simulink model "UnusedModels"  (R2015a)
settings: Solver=ode45  StartTime=0.0  StopTime=10.0  RelTol=1e-3
values from neighbouring files (symbols this model uses):
  car_params = Simulink_Car_params    [TV2016_parameters.m]
  energyLimitControl = Simulink_energyLimit    [TV2016_parameters.m]
  settings = Simulink_Settings    [TV2016_parameters.m]
  speedEstimation = Simulink_speedEst    [TV2016_parameters.m]
  tractionControl = Simulink_tc    [TV2016_parameters.m]
  yawRateControl = Simulink_yawRate    [TV2016_parameters.m]
undefined symbols (not defined in the file or in its folder): canChannel, Use_Estimated_velocity
libraries: canlib x44, CarMaker4SL x33, canmsglib x28, simulink x6
(part 4 of 4)

== matlab function UnusedModels/MATLAB Function ==
  data: Mz_ref input; Fx input; states input; Ti_lim output Bus: Ti_lim; Mz_error output; CM_Fxy input; car_params parameter; yaw_acc input; settings parameter; Mz output; R_eff_i input; Ti_prev input; Mz_calc output; Fz_ratio output; Fzi output; Long output; PseudoError output
function [Ti_lim, Mz_error,Mz,Mz_calc,Fz_ratio,Fzi,Long,PseudoError]= fcn(Mz_ref,Fx, states, CM_Fxy, car_params,yaw_acc,settings, R_eff_i, Ti_prev)
%#codegen


% % Splitte opp foran og bak-> vil hindre negativt moment på ytterhjul
% 
% %Fz scaling factor Calculation
% %The thought is 0 N Fz -> Cant use this wheel for torque
% % < 400N Fz , can use this wheel fully
% %Tire forces..
% Fzi = [states.Input_Fz_FL states.Input_Fz_FR states.Input_Fz_RL states.Input_Fz_RR]';
% 
% for i=1:4
%     if Fzi(i) <= 0
%         Fzi(i) = 1;
%     end
% end
% 
% dDt_Fz = 1/400;
% Fzi_Scaling = Fzi*dDt_Fz;
% for i=1:4
%     if ( Fzi_Scaling(i) < 0 )
%         Fzi_Scaling(i) = 0;
%     elseif (Fzi_Scaling(i) > 1)
%         Fzi_Scaling(i) = 1;
%     end
% end
% % 
% % % Scale all wheels with Fz first 
% % F_all = zeros(1,4);
% % %F_all = prod([Fx/4 Fx/4 Fx/4 Fx/4; Fzi_Scaling']);
% % F_all =[Fx/4 Fx/4 Fx/4 Fx/4];
% % % Find lateral split ratio
% % % Find longitudinal split ratio
% % 
% % if ((abs(r_ref)-abs(states.r)) <= 0)
% %     %Oversteering. Reduce torque on outer wheels
% %     ow_sf = 1- (1/settings.yaw_control_max_moment)*abs(Mz_ref);
% %     if sign(r_ref) == -1 
% %         %Right turn 
% %         F_all = prod([F_all;ow_sf 1 ow_sf 1]);
% %     else
% %         %Left turn
% %         F_all = prod([F_all;1 ow_sf 1 ow_sf]);
% %     end
% % else 
% %     %Find lateral split ratio
% %     l_sr = (1/settings.yaw_control_max_moment)*abs(Mz_ref);
% %     if sign(r_ref) == -1
% %         %Right turn
% %         F_all = prod([F_all;l_sr,(1-l_sr), l_sr, (1-l_sr)]);
% %     else 
% %         F_all = prod([F_all; (1-l_sr), l_sr , (1-l_sr) l_sr]);
% %     end
% % end
% 
% %Ratio between left and right wheels
% % Cases. 
% % 1. left turn r_ref larger than r. split more to outer wheels
% % 2. left turn r larger than r_ref. Reduce outher wheel torque
%     % Make scaling factor for outer wheels to reduce torque based on the Mz
% 
% % 3. right turn r_ref larger than r. split more to outer wheels
% % 4. right turn r larger than r_ref. Reduce outher wheel torque
%      % Make scaling factor for outer wheels to reduce torque based on the Mz
% 
% 
% 
% 
% %Calculate attainable torque for each motor
% Eng_rot_all = [Eng_rot.Eng_rot_FL Eng_rot.Eng_rot_FR Eng_rot.Eng_rot_RL Eng_rot.Eng_rot_RR];
% T_m_max = zeros(4,1);
% b = 20;
% a = -1/1000;
% x0 = 14000;
% for i=1:4
%     if Eng_rot_all(i) > 14000
%         T_m_max(i) = a*(Eng_rot_all(i)-x0) + b;
%     else 
%         T_m_max(i) = 21;
%     end
% end
% %Calculate allowable negative Torque limit
% T_m_neg = zeros(4,1);
% for i=1:4
%     if Fx == 0
%         T_m_neg(i) = 0;
%     elseif sign(Mz_ref) == sign(states.FL_Whl_Ang)
%         T_m_neg(i) = 0;
%     end
%     % Legge til at innerdekk ikke kan bruke negative torque eller positive
% end
% 
% 
% %1 = FL, 2 = FR, 3 = RL , 4 = RR
% R = [R_eff_i.R_FL; R_eff_i.R_FR ; R_eff_i.R_RL ; R_eff_i.R_RR]';
% 
% S = (states.FL_Whl_Ang + states.FR_Whl_Ang) / 2;
% l1 = car_params.t_f*cos(S) - car_params.l_f*sin(S);
% l2 = car_params.t_f*cos(S) + car_params.l_f*sin(S);
% l3 = car_params.t_r;
% l4 = car_params.t_r;
% 
% L = [-l1; l2; -l3; l4];  %*0.8;
% L_scaled = prod( [L'; Fzi'*settings.mui]);
% Tot_torque_scaled = prod( [1 1 1 1;Fzi'*settings.mui]);
% A_o = [L'; 1   1    1  1];
% %A = A*diag([Fzi'*settings.mui]);
% 
% %A = [L_scaled;Tot_torque_scaled]; %
% A = [L_scaled;Tot_torque_scaled
%     ]; % 
% 
% 
% %A_sat = diag([1 1 1 1]);
% 
% b = [Mz_ref; Fx];
% %Wu = diag([Fzi'*settings.mui]);
% Wu = diag( [1/Fzi(1)^2 1/Fzi(2)^2  1/Fzi(3)^2  1/Fzi(4)^2]);
%     
% 
%  
% Fx_i = zeros(4,1);
% %x is weighted by input
% %Fx_i = pinv(A)*b; %
% 
% 
% %Weighting by external weight matrix
% %Fx_i = Wu\(pinv(A/Wu))*b;
% Fx_i = inv(Wu)*A'*(inv(A*inv(Wu)*A'))*b
% %Fx_i = prod( [(pinv(A)*b)';Fzi_Scaling' ])';
% %Fx_i = (pinv(A)*b)
% PseudoError = A*Fx_i - b;
% Long = Tot_torque_scaled*Fx_i;
% 
% %x = (0,1)
% %Allocation based on Fz*x
% Ti_all = prod([Fx_i';R; Fzi'*settings.mui])*(1/settings.gear_ratio);
% Ti_lim_struct = struct;
% Ti_lim_struct.T_FL = Ti_all(1);
% Ti_lim_struct.T_FR = Ti_all(2);
% Ti_lim_struct.T_RR = Ti_all(4);
% Ti_lim_struct.T_RL = Ti_all(3);
% 
% 
% % Ti_all = prod([Fx_i';R])*(1/settings.gear_ratio)
% % Ti_lim_struct = struct;
% % Ti_lim_struct.T_FL = Ti_all(1);
% % Ti_lim_struct.T_FR = Ti_all(2);
% % Ti_lim_struct.T_RR = Ti_all(4);
% % Ti_lim_struct.T_RL = Ti_all(3);
% 
% Ti_lim = Ti_lim_struct; 
% 
% %Mz = -car_params.Iz * yaw_acc ; This is the total yaw moment which is not
% %what i am after.
% Mz = single(0); 
% Mz_calc = L_scaled*Fx_i;
% Mz_error = Mz_ref - Mz_calc;
% Fz_ratio = zeros(4,1);
% 
% for i=1:4
%     Fz_ratio(i,1) = sum( settings.mui^2*Fzi.^2 - Fx_i.^2) / (settings.mui^2*Fzi(i)^2 - Fx_i(i)^2);
% end

 
 %------------------------------------------------------------------------
 %------------------- Split Front/Rear------------------------------------
 %------------------------------------------------------------------------
 
% Splitte opp foran og bak-> vil hindre negativt moment på ytterhjul

%Fz scaling factor Calculation
%The thought is 0 N Fz -> Cant use this wheel for torque
% < 400N Fz , can use this wheel fully
%Tire forces..
Fzi = [states.Fz_FL states.Fz_FR states.Fz_RL states.Fz_RR]';

for i=1:4
    if Fzi(i) <= 0
        Fzi(i) = 1;
    end
end

dDt_Fz = 1/400;
Fzi_Scaling = Fzi*dDt_Fz;
for i=1:4
    if ( Fzi_Scaling(i) < 0 )
        Fzi_Scaling(i) = 0;
    elseif (Fzi_Scaling(i) > 1)
        Fzi_Scaling(i) = 1;
    end
end

%Calculate attainable torque for each motor
motor_RPMS = [states.RPM_FL states.RPM_FR  states.RPM_RL  states.RPM_RL]; 
T_m_max = zeros(4,1);
b = 20;
a = -1/1000;
x0 = 14000;
for i=1:4
    if motor_RPMS(i) > 14000
        T_m_max(i) = a*(motor_RPMS(i)-x0) + b;
    else 
        T_m_max(i) = 21;
    end
end
%Calculate allowable negative Torque limit
T_m_neg = zeros(4,1);
for i=1:4
    if Fx == 0
        T_m_neg(i) = 0;
    elseif sign(Mz_ref) == sign(states.FL_Whl_Ang)
        T_m_neg(i) = 0;
    end
    % Legge til at innerdekk ikke kan bruke negative torque eller positive
end


%1 = FL, 2 = FR, 3 = RL , 4 = RR
R = [R_eff_i.R_FL; R_eff_i.R_FR ; R_eff_i.R_RL ; R_eff_i.R_RR]';

S = (states.FL_Whl_Ang + states.FR_Whl_Ang) / 2;
l1 = car_params.t_f*cos(S) - car_params.l_f*sin(S); 
l2 = car_params.t_f*cos(S) + car_params.l_f*sin(S);
l3 = car_params.t_r;
l4 = car_params.t_r;

L = [-l1; l2; -l3; l4];  %*0.8;
L_scaled = prod( [L'; Fzi'*settings.mui]);
Tot_torque_scaled = prod( [1 1 1 1;Fzi'*settings.mui]);
A = [L_scaled;Tot_torque_scaled]; % 

A_f = [L_scaled(1) L_scaled(2);Tot_torque_scaled(1) Tot_torque_scaled(2)];
A_r = [L_scaled(3) L_scaled(4);Tot_torque_scaled(3) Tot_torque_scaled(4)];
%alfa_r = 0.5;

alfa_r =  (Fzi(3) + Fzi(4)) / (Fzi(1) + Fzi(2) +Fzi(3) + Fzi(4)); % How much of fz is at the rear..
b_f = [ (1-alfa_r) * Mz_ref; (1-alfa_r)*Fx];
b_r = [alfa_r*Mz_ref; alfa_r*Fx]; 


b = [Mz_ref; Fx];
%Wu = diag( [1/Fzi(1)^2 1/Fzi(2)^2  1/Fzi(3)^2  1/Fzi(4)^2]);
Wu_f = diag( [1/Fzi(1)^2 1/Fzi(2)^2]);
Wu_r = diag( [1/Fzi(3)^2 1/Fzi(4)^2]);

%u_f = zeros(2,1); % [-1,1] if over then it is saturated
%u_r = zeros(2,1); % [-1,1] 

Fx_i = zeros(4,1);
%x is weighted by input
%Fx_i = pinv(A)*b; %

%Weighting by external weight matrix
%Fx_i = Wu\(pinv(A/Wu))*b;

% u_f = Wu_f\pinv(A_f/Wu_f)*b_f
u_f2 = pinv(A_f)*b_f;
% u_r = Wu_r\pinv(A_r/Wu_r)*b_r;



%u_f = daisy_MzTot(u_f_pre,A_f,b_f,Wu_f);
%u_r = daisy_MzTot(u_r_pre,A_r,b_r,Wu_r);

% If sign(Mz) != turn allow negative torques for outer wheels
% Maybe if too high yaw rate only minimize Mz error.
% If not just use mz + tot(all positive)


% TRY THIS &
% Least squares for only Mz
% Then increase torque until saturation. But increase in which direction ?
A_mz_f = [A(1,1) A(1,2)];
A_mz_r = [A(1,3) A(1,4)];
b_mz_f = (1-alfa_r)*Mz_ref;
b_mz_r = alfa_r*Mz_ref;
u_f = single([0;0]);
u_r = single([0;0]);


u_f = distPseudoIterative_2State(A_f, b_f, states.r);
u_r = distPseudoIterative_2State(A_r, b_r, states.r);

%-------------------------------------------------%
%-----------Determine torque setpoints---------------%
%-------------------------------------------------%
Ti_all = prod([u_f' u_r';R; Fzi'*settings.mui])*(1/settings.gear_ratio);


Ti_lim_struct = struct;
Ti_lim_struct.T_FL = Ti_all(1);
Ti_lim_struct.T_FR = Ti_all(2);
Ti_lim_struct.T_RR = Ti_all(4);
Ti_lim_struct.T_RL = Ti_all(3);

Ti_lim = Ti_lim_struct; 



% if ( sign(Mz_ref) ~= sign(states.r) ) && abs(Mz_ref) > 30 && abs(states.r) > 1.3
% else
%     u_f = distPseudoIterative_2State(A_f, b_f, states.r);
%     u_r = distPseudoIterative_2State(A_r, b_r, states.r);
% end


% if one element of u_f is absolute > 1. 
% Find out which
% If only one, then saturate that input and solve equation for the other
% one.
% If that one saturates as well Finish (for now)
% If both saturated Finish (for now)


%u_f = inv(Wu_f)*A_f'*(inv(A_f*inv(Wu_f)*A_f'))*b_f;
%u_r = inv(Wu_r)*A_r'*(inv(A_r*inv(Wu_r)*A_r'))*b_r;


%-----------------------------------
%-------Allokering med vekt artikkel---

u_opt_f = (Wu_f + A_f'*A_f)\A_f'*b_f;
%u_f = [0;0];
%u_f = pinv(A_f)*b_f;
%u_r = pinv(A_r)*b_r

%Fx_i = inv(Wu)*A'*(inv(A*inv(Wu)*A'))*b
%Fx_i = prod( [(pinv(A)*b)';Fzi_Scaling' ])';
%Fx_i = (pinv(A)*b)

%x = (0,1)
%Allocation based on Fz*x


%Ti_all = prod([Fx_i';R; Fzi'*settings.mui])*(1/settings.gear_ratio);





%Mz = -car_params.Iz * yaw_acc ; This is the total yaw moment which is not
%what i am after.

PseudoError = single(0); % A*Fx_i - b;
Long = single(0); % Tot_torque_scaled*Fx_i;

Mz = single(0); 
Mz_calc = L_scaled*[u_f;u_r];
Mz_error = Mz_ref - Mz_calc;
%Mcalc = L'*(prod([Ti_all';1./R])*GR)';
%Mz_error = Mz_ref - Mcalc;

Fz_ratio = zeros(4,1);

for i=1:4
    Fz_ratio(i,1) = sum( settings.mui^2*Fzi.^2 - Fx_i.^2) / (settings.mui^2*Fzi(i)^2 - Fx_i(i)^2);
end
end


function u_x = daisy_Mz(u_in,A,b)
    u_x = single(zeros(2,1));
    l = u_in(1);
    r = u_in(2);
    if ( abs(l) > 1) && ( abs(r) <= 1) 
        %W = W(2,2); % Second input should be weighted
        A_x = A(1,2)
        b_new = b - sign(l)*A(1,1);
        r = pinv(A_x)*b_new;
        l = 1*sign(l);
        u_x = [l;r];
    elseif ( abs(r) > 1) && ( abs(l) <= 1)
        %W = W(1,1); % First input should be weighted
        A_x = A(1,1);
        b
        b_new = b - sign(r)*A(1,2)
        l = pinv(A_x)*b_new
        r = 1*sign(r)
        u_x = [l;r]
        error = A*u_x - b    
        % Kommer ut av daisy med negativ torque på ene hjulet-> vanlig
        % pseudo liker det dårlig( fx + fx = tot_fx).. blir ustabilt.
    elseif ( abs(r) > 1) && ( abs(l) > 1)
        %Solve for both, then choose the best
        
        u_x = [sign(l);sign(r)];
        
        hoi = 5
    else 
        u_x = u_in;
    end
end

function u = distPseudoIterative(B_in, tau,nr_u_solved,u_size)
    % B = A, tau = b
    coder.varsize('B',[2,4]);
    coder.varsize('u_sat',[4,1]);
    coder.varsize('B_sat',[2,4]);
    coder.varsize('B_unsat',[2,4]);
    B = B_in;
    u_solved = single(-10*ones(u_size,1));
%     u_sat   = zeros(4,1);
%     B_sat   = zeros(2, 4);
%     B_unsat = zeros(2, 4);
    for z=1:10
        z
        [row_B,col_B] = size(B);
        row_tau = row_B;
        u_1 = pinv(B)*tau
        %Find number of saturated elements
        nr_sat_elements = 0;
        for i=1:col_B
            if abs(u_1(i)) > 1
                nr_sat_elements = nr_sat_elements + 1;
            end
        end
        if (nr_sat_elements == 0) 
            open_spot_counter = 0;
            % Must fill in u_1 into u_solved...
            if nr_u_solved == 0
                % If solved on first attempt fit u_1 into u solved and
                % return
                u = u_1;
                return  
            else
                % Not first attempt, then need to fill in u_1 into u_solved
                for i=1:size(u_1,1)
                    for a=1:u_size
                        if u_solved(a) == -10
                            open_spot_counter = open_spot_counter + 1;
                            if open_spot_counter == i 
                                u_solved(a) = sign(u_1(i));
                                break
                            end
                        end
                    end
                end   
                u = u_solved;
                return
            end   
        end
        %Split into saturated and non saturated
        
%         if (nr_sat_elements == 1)
%             u_sat = 0;
%             B_sat = zeros(row_B,1);
%             B_unsat = zeros(row_B, col_B - 1);
%         elseif (nr_sat_elements == 2)
%             u_sat = zeros(2,1);
%             B_sat = zeros(row_B,2);
%             B_unsat = zeros(row_B, col_B - 2);
% 
%         elseif (nr_sat_elements == 3)
%             u_sat = zeros(3,1);
%             B_sat = zeros(row_B,3);
%             B_unsat = zeros(row_B, col_B - 3);
% 
%         elseif (nr_sat_elements == 4)
%             u_sat = zeros(4,1);
%             B_sat = zeros(row_B,4); 
%             B_unsat = zeros(1,1);
% 
%         else
%             B = zeros(row_B,1);
%             u_sat = 0;
%             B_sat = zeros(row_B,1); 
%         end
        
        assert(nr_sat_elements < 5);
        u_sat   = zeros(nr_sat_elements,1);
        B_sat   = zeros(row_B, nr_sat_elements);
        B_unsat = zeros(row_B, col_B - nr_sat_elements);
        sat_counter     = 1;
        unsat_counter   = 1;
        open_spot_counter = 0;
        for i=1:col_B
            if abs(u_1(i)) > 1
                u_sat(sat_counter) = sign(u_1(i));
                %Fill in new saturated elements into the solution vector
                % Need to add the elements
                if col_B == u_size
                    u_solved(i) = sign(u_1(i));
                else              
                    %Search for first open spot corresponding with i
                    for a=1:u_size
                        if u_solved(a) == -10
                            open_spot_counter = open_spot_counter + 1;
                            if open_spot_counter == i 
                                u_solved(a) = sign(u_1(i))
                                break
                            end
                            
                        end
                    end
                end
                
                nr_u_solved = nr_u_solved + 1;
                for j=1:row_B
                    B_sat(j, sat_counter) = B(j,i);
                end  
                sat_counter = sat_counter + 1;
            elseif abs(u_1(i)) <= 1
                for j=1:row_B
                    B_unsat(j, unsat_counter) = B(j,i);
                end
                unsat_counter = unsat_counter + 1;
            else
                thisShouldNotHappen = 1
            end

        end
        % Now I have saturated B and u and unsaturated B
        tau = tau - B_sat*u_sat;
        B = single(B_sat);
%         B = zeros(size(B_sat,1),size(B_sat,2))
%         for i=1:size(B_sat,1)
%             for j=1:size(B_sat,2)
%                 B(i,j) = B_sat(i,j);
%             end
%         end
        
        %Now I have the new problem
        if nr_u_solved == u_size 
            u = u_solved;
            return
        end
    end
    u = u_solved;
end
    



function u_x = daisy_MzTot(u_in,A,b,W)
    u_x = single(zeros(2,1));
    l = u_in(1);
    r = u_in(2);
    if ( abs(l) > 1) & ( abs(r) <= 1) 
        W = W(2,2); % Second input should be weighted
        A_x = [ A(1,2);A(2,2)];
        b_new = b - sign(l)*[A(1,1);A(2,1)];
        r = pinv(A_x)*b_new;
        l = 1*sign(l);
        u_x = [l;r];
    elseif ( abs(r) > 1) & ( abs(l) <= 1)
        W = W(1,1); % First input should be weighted
        A_x = [ A(1,1);A(2,1)]
        b
        b_new = b - sign(r)*[A(1,2);A(2,2)]
        l = pinv(A_x)*b_new
        r = 1*sign(r)
        u_x = [l;r]
        error = A*u_x - b    
        % Kommer ut av daisy med negativ torque på ene hjulet-> vanlig
        % pseudo liker det dårlig( fx + fx = tot_fx).. blir ustabilt.
    elseif ( abs(r) > 1) & ( abs(l) > 1)
        %Solve for both, then choose the best
        u_x = [sign(l); sign(r)]
        hoi = 5
    else 
        u_x = u_in;
    end
end
%u_f = Wu_f\pinv(A_f/Wu_f)*b_f

function u = distPseudoIterative_2State(B, tau, r)
    u_1 = pinv(B)*tau;
    if ( abs(u_1(1)) <= 1 && abs(u_1(2)) <= 1 )
        % None saturated. Return
        u = u_1;
        return
    elseif ( abs(u_1(1)) > 1 && abs(u_1(2)) <= 1 )
        % Nr 1 saturated
        B_sat = [B(1,1);B(2,1)];
        B_unsat = [B(1,2);B(2,2)];
        tau_proj = tau - B_sat*(sign(u_1(1)));
        right = pinv(B_unsat)*tau_proj;
        if abs(right) > 1 
            right = sign(right);
        end

        u = [sign(u_1(1));right]; 
        % Do something if u is also saturated
        return

    elseif ( abs(u_1(1)) <= 1 && abs(u_1(2)) > 1 )
         % Nr 2 saturated
        B_sat = [B(1,2);B(2,2)];
        B_unsat = [B(1,1);B(2,1)];
        tau_proj = tau - B_sat*(sign(u_1(2)));
        left = pinv(B_unsat)*tau_proj;
        if abs(left) > 1 
            left = sign(left);
        end   
        u = [left;sign(u_1(2))]; 
        % Do something if u is also saturated
        return

    elseif ( abs(u_1(1)) > 1 && abs(u_1(2)) > 1 )
        % If turning right input 1 should be saturated and input 2
        % recomputed
        %If turning left opposite

        if ( sign(r) == 1)
            %turning left, right wheel saturate
            B_sat = [B(1,2);B(2,2)];
            B_unsat = [B(1,1);B(2,1)];
            tau_proj = tau - B_sat*(sign(u_1(2)));
            left = pinv(B_unsat)*tau_proj;
            if abs(left) > 1 
                left = sign(left);
            end   
            u = [left;sign(u_1(2))];
            return
        elseif (sign(r) == -1)
            %turning right
            % Nr 1 saturated
            B_sat = [B(1,1);B(2,1)];
            B_unsat = [B(1,2);B(2,2)];  
            tau_proj = tau - B_sat*(sign(u_1(1)));
            right = pinv(B_unsat)*tau_proj;
            if abs(right) > 1 
                right = sign(right);
            end
            u = [sign(u_1(1));right]; 
            % Do something if u is also saturated
            return
        else
            %Not turning
            %Saturate both and return
            u = [sign(u_1(1));sign(u_1(2))];  
            return
        end
    else
        u = u_1;
        return
    end
end

== matlab function UnusedModels/Estimations /RPM to wheel x velocities/Calculate velocity of each wheel ==
  data: sensor input; Whl_v_FL output; Whl_v_FR output; Whl_v_RL output; Whl_v_RR output; settings parameter; car_params parameter
function [Whl_v_FL, Whl_v_FR, Whl_v_RL, Whl_v_RR]  = RpmToVelocity(sensor,settings,car_params)
%#codegen

%Conversion from RPM to rad/s for the wheel
c = single(2*pi/(car_params.GR*60));

% Simple atm. Not considering rotation and vy
Whl_v_FL = sensor.RPM_FL*c*car_params.r_eff;
Whl_v_FR = sensor.RPM_FR*c*car_params.r_eff;
Whl_v_RL = sensor.RPM_RL*c*car_params.r_eff;
Whl_v_RR = sensor.RPM_RR*c*car_params.r_eff;

== matlab function UnusedModels/SimpleTv/MATLAB Function ==
  data: muR input; Ti_lim output Bus: Ti_lim; Fx input; states input; settings parameter; R_eff_i input; car_params parameter; Mz_ref input; Ti_max output; Mz_error output
function [Ti_lim,Ti_max,Mz_error]  = fcn(muR,Fx,states,settings,R_eff_i, car_params,Mz_ref )
%#codegen
%STATES
r = states.r;

%PARAMETERS
mu = settings.mui;
tf = car_params.t_f*2;
tr = car_params.t_r*2;
GR = car_params.GR;
R = [R_eff_i.R_FL; R_eff_i.R_FR ; R_eff_i.R_RL ; R_eff_i.R_RR]';
%Load Transfer
Fzi = [states.Fz_FL states.Fz_FR states.Fz_RL states.Fz_RR]';
alfa_r =  (Fzi(3) + Fzi(4)) / (Fzi(1) + Fzi(2) +Fzi(3) + Fzi(4)); 






%FIND MAXIMUM ALLOWED MOTOR TORQUE, TIRE/MOTOR
Ti_max          = single(zeros(4,1));
Ti_max_tire     = single(zeros(4,1));
Ti_max_motor    = single(zeros(4,1));

RPM = [states.RPM_FL, states.RPM_FR, states.RPM_RL, states.RPM_RR];
a = 8/7000;
a2 = 13/1000;
for i=1:4
    if RPM(i) >= 20000 
        Ti_max_motor(i) = 0;
    elseif RPM(i) > 12000 & RPM(i) < 19000
        Ti_max_motor(i) = -a*(RPM(i) - 12000) + 21;
    elseif RPM(i) > 19000 & RPM(i) < 20000
        Ti_max_motor(i) = -a2*(RPM(i) - 19000) + 13;
    else 
        Ti_max_motor(i) = 21;
    end
end
%Tire saturation based on mu and Fz
for i=1:4
    Ti_max_tire(i) = Fzi(i)*mu*R(i)/GR;
end
% Find minimum of tire saturation Torque and motor
for i=1:4
    Ti_max(i) = min(Ti_max_tire(i), Ti_max_motor(i));
end
%**********************************************%

T_F = single(zeros(2,1));
T_R = single(zeros(2,1));

T_F = dist(Ti_max(1), Ti_max(2), Fx, R(1), R(2), (1-alfa_r), Mz_ref, GR, tf);
T_R = dist(Ti_max(3), Ti_max(4), Fx, R(3), R(4), alfa_r, Mz_ref, GR, tr);


% T_FL = (1-alfa_r)*Fx*R(1)/(2*GR) - (1-alfa_r)*Mz_ref*R(1)/(GR*tf);
% T_FR = (1-alfa_r)*Fx*R(2)/(2*GR) + (1-alfa_r)*Mz_ref*R(2)/(GR*tf);
% T_RL = (alfa_r)*Fx*R(3)/(2*GR) - alfa_r*Mz_ref*R(3)/(GR*tr);
% T_RR = (alfa_r)*Fx*R(4)/(2*GR) + alfa_r*Mz_ref*R(4)/(GR*tr);

%Ti_all = [T_FL, T_FR, T_RL, T_RR];
Ti_all = [T_F' T_R'];

Ti_lim_struct = struct;
Ti_lim_struct.T_FL = Ti_all(1);
Ti_lim_struct.T_FR = Ti_all(2);
Ti_lim_struct.T_RR = Ti_all(4);
Ti_lim_struct.T_RL = Ti_all(3);

Ti_lim = Ti_lim_struct;



% Mz_error Calc

S = states.steering_angle;
l1 = car_params.t_f*cos(S) - car_params.l_f*sin(S); 
l2 = car_params.t_f*cos(S) + car_params.l_f*sin(S);
l3 = car_params.t_r;
l4 = car_params.t_r;

L = [-l1; l2; -l3; l4];
Fx_all = prod([Ti_all; 1./R;])*GR;
Mz_allocated = L'*Fx_all';
Mz_error = Mz_ref - Mz_allocated;


end

function T = dist(L_max, R_max, Fx, R_eff_L, R_eff_R, alfa, Mz_ref, GR, t )
    T = single(zeros(2,1));
    L = alfa*Fx*R_eff_L/(2*GR) - alfa*Mz_ref*R_eff_L/(GR*t);
    R = alfa*Fx*R_eff_R/(2*GR) + alfa*Mz_ref*R_eff_R/(GR*t);

    if ( abs(L) <=  L_max) && ( abs(R) <= R_max)
        % None are saturated. Return
        T = [L;R];
        return
    elseif abs(L) > L_max && abs(R) < R_max
        % Left is saturated
        % How much?
        Sat_amount = abs(L) - L_max;
        L = L - sign(L)*Sat_amount;
        R = R - sign(R)*Sat_amount;
        T = [L;R];
        return;
    elseif abs(R) > R_max && abs(L) < L_max
        Sat_amount = abs(R) - R_max;
        L = L - sign(L)*Sat_amount;
        R = R - sign(R)*Sat_amount;
        T = [L;R];
        return;
    elseif (abs(R) > R_max) && (abs(L) > L_max)
        %Which is the most saturated?
        Sat_amount = max( (abs(L) - L_max), (abs(R)- R_max));
        L = L - sign(L)*Sat_amount;
        R = R - sign(R)*Sat_amount;
        T = [L;R];
        return;
    else
        T = [L;R];
        return
    end
end

== matlab function UnusedModels/Function-Call Subsystem/MATLAB Function ==
  data: trq_pos_16 input; trq_pos_f output; trq_neg_16 input; w_set_16 input; trq_neg_f output; w_set_f output; settings parameter
function [trq_pos_f, trq_neg_f, w_set_f] = fcn(trq_pos_16, trq_neg_16, w_set_16, settings)
%#codegen

Sf = settings.scaling_factor;
trq_pos_f = double( trq_pos_16/Sf);
trq_neg_f = double( trq_neg_16/Sf);
w_set_f = double( w_set_16);

== matlab function UnusedModels/Estimations /Normal Force Direct Calculation/MATLAB Function ==
  data: sensor input; settings parameter; car_params parameter; Fz_FL output; Fz_FR output; Fz_RL output; Fz_RR output
function [Fz_FL, Fz_FR, Fz_RL, Fz_RR] = normalForceEstimation(sensor, settings,car_params)
%#codegen

te = settings.control_system_sample_time;
ms = car_params.sprung_mass; 
mv = car_params.mass; % Total mass( driver + car)
l = car_params.l; %Wheel base
lr = car_params.l_r;
lf = car_params.l_f;
hr = car_params.h_r;
hf = car_params.h_f;
tf = car_params.t_f*2; % Front track
tr = car_params.t_r*2; % Rear track
kf = car_params.roll_stiff_f;
kr = car_params.roll_stiff_r;
Ixx = car_params.Ixx;
hcr = car_params.h_cr;
Kr = car_params.K_r;
Cr = car_params.C_r;
hc = car_params.CoG_height;
g = 9.81;

ax = sensor.ax;
ay = sensor.ay;

Fz_FL = 0.5*mv*(lr*g/l - hc*ax/l) - mv*(lr*g/l - hc*ax/l) * hc*ay/(tf*g);

Fz_FR = 0.5*mv*(lr*g/l - hc*ax/l) + mv*(lr*g/l - hc*ax/l) * hc*ay/(tf*g);

Fz_RL = 0.5*mv*(lf*g/l + hc*ax/l) - mv*(lf*g/l + hc*ax/l) * hc*ay/(tr*g);

Fz_RR = 0.5*mv*(lf*g/l + hc*ax/l) + mv*(lf*g/l + hc*ax/l) * hc*ay/(tr*g);




end

== matlab function UnusedModels/Function-Call Subsystem1/MATLAB Function1 ==
  data: trq_pos_16 input; trq_pos_f output; trq_neg_16 input; w_set_16 input; trq_neg_f output; w_set_f output; settings parameter
function [trq_pos_f, trq_neg_f, w_set_f] = fcn(trq_pos_16, trq_neg_16, w_set_16, settings)
%#codegen

Sf = settings.scaling_factor;
trq_pos_f = double( trq_pos_16/Sf);
trq_neg_f = double( trq_neg_16/Sf);
w_set_f = double( w_set_16);

== matlab function UnusedModels/Function-Call Subsystem3/MATLAB Function3 ==
  data: trq_pos_16 input; trq_pos_f output; trq_neg_16 input; w_set_16 input; trq_neg_f output; w_set_f output; settings parameter
function [trq_pos_f, trq_neg_f, w_set_f] = fcn(trq_pos_16, trq_neg_16, w_set_16, settings)
%#codegen

Sf = settings.scaling_factor;
trq_pos_f = double( trq_pos_16/Sf);
trq_neg_f = double( trq_neg_16/Sf);
w_set_f = double( w_set_16);

== matlab function UnusedModels/Function-Call Subsystem2/MATLAB Function2 ==
  data: trq_pos_16 input; trq_pos_f output; trq_neg_16 input; w_set_16 input; trq_neg_f output; w_set_f output; settings parameter
function [trq_pos_f, trq_neg_f, w_set_f] = fcn(trq_pos_16, trq_neg_16, w_set_16, settings)
%#codegen

Sf = settings.scaling_factor;
trq_pos_f = double( trq_pos_16/Sf);
trq_neg_f = double( trq_neg_16/Sf);
w_set_f = double( w_set_16);

== matlab function UnusedModels/Estimations /Subsystem/Compute Derivative of RPM ==
  data: RPM_FL input; rateRPM_FL output; RPM_FR input; RPM_RL input; RPM_RR input; settings parameter; rateRPM_FR output; rateRPM_RL output; rateRPM_RR output
function [rateRPM_FL,rateRPM_FR,rateRPM_RL,rateRPM_RR]...
          = computeRPMDerivative(RPM_FL,RPM_FR,RPM_RL,RPM_RR,settings)
%#codegen

t = settings.control_system_sample_time;
sg_Weight = single( [ -1; 8; 0; -8; 1] );

nr_Coefficients = uint32(5);
persistent firstIteration;
persistent frame;
persistent RPM_prev_FL;
persistent RPM_prev_FR;
persistent RPM_prev_RL;
persistent RPM_prev_RR;


if isempty(firstIteration)
        firstIteration = 2;
        RPM_prev_FL = RPM_FL;
        RPM_prev_FR = RPM_FR;
        RPM_prev_RL = RPM_RL;
        RPM_prev_RR = RPM_RR;
        
        frame = single(zeros(1,nr_Coefficients));
        rateRPM_FL = single(0);
        rateRPM_FR = single(0);
        rateRPM_RL = single(0);
        rateRPM_RR = single(0);
else
    rateRPM_FL = abs( (RPM_FL - RPM_prev_FL)/(t));
    rateRPM_FR = abs( (RPM_FR - RPM_prev_FR)/(t));
    rateRPM_RL = abs( (RPM_RL - RPM_prev_RL)/(t));
    rateRPM_RR = abs( (RPM_RR - RPM_prev_RR)/(t));
    RPM_prev_FL = RPM_FL;
    RPM_prev_FR = RPM_FR;
    RPM_prev_RL = RPM_RL;
    RPM_prev_RR = RPM_RR;
    
    
%     frame = [RPM, frame(1:(end-1))]    
%     %Calculate output
%     rateRPM = abs((frame*weight_Vector)./(12*ts));


end

== matlab function UnusedModels/Function-Call Subsystem4/MATLAB Function ==
  data: trq_pos_16 input; trq_pos_f output; trq_neg_16 input; w_set_16 input; trq_neg_f output; w_set_f output; settings parameter
function [trq_pos_f, trq_neg_f, w_set_f] = fcn(trq_pos_16, trq_neg_16, w_set_16, settings)
%#codegen

Sf = settings.scaling_factor;
trq_pos_f = double( trq_pos_16/Sf);
trq_neg_f = double( trq_neg_16/Sf);
w_set_f = double( w_set_16);

== matlab function UnusedModels/Function-Call Subsystem4/MATLAB Function1 ==
  data: trq_pos_16 input; trq_pos_f output; trq_neg_16 input; w_set_16 input; trq_neg_f output; w_set_f output; settings parameter
function [trq_pos_f, trq_neg_f, w_set_f] = fcn(trq_pos_16, trq_neg_16, w_set_16, settings)
%#codegen

Sf = settings.scaling_factor;
trq_pos_f = double( trq_pos_16/Sf);
trq_neg_f = double( trq_neg_16/Sf);
w_set_f = double( w_set_16);

== matlab function UnusedModels/Function-Call Subsystem4/MATLAB Function2 ==
  data: trq_pos_16 input; trq_pos_f output; trq_neg_16 input; w_set_16 input; trq_neg_f output; w_set_f output; settings parameter
function [trq_pos_f, trq_neg_f, w_set_f] = fcn(trq_pos_16, trq_neg_16, w_set_16, settings)
%#codegen

Sf = settings.scaling_factor;
trq_pos_f = double( trq_pos_16/Sf);
trq_neg_f = double( trq_neg_16/Sf);
w_set_f = double( w_set_16);

== matlab function UnusedModels/Function-Call Subsystem4/MATLAB Function3 ==
  data: trq_pos_16 input; trq_pos_f output; trq_neg_16 input; w_set_16 input; trq_neg_f output; w_set_f output; settings parameter
function [trq_pos_f, trq_neg_f, w_set_f] = fcn(trq_pos_16, trq_neg_16, w_set_16, settings)
%#codegen

Sf = settings.scaling_factor;
trq_pos_f = double( trq_pos_16/Sf);
trq_neg_f = double( trq_neg_16/Sf);
w_set_f = double( w_set_16);

== matlab function UnusedModels/Fz_Estimation/FzEst ==
  data: normalForces output Bus: normalForces; sensor input; settings parameter; car_params parameter; x_out output; xv_out output; FZ output; delta_Fzl output
function [normalForces, x_out,xv_out,FZ,delta_Fzl] = normalForceEstimation(sensor, settings,car_params)
%#codegen

te = settings.control_system_sample_time;

ms = car_params.sprung_mass; 
mv = car_params.mass; % Total mass( driver + car)
l = car_params.l; %Wheel base
lr = car_params.l_r;
lf = car_params.l_f;
hr = car_params.h_r;
hf = car_params.h_f;
ef = car_params.t_f*2; % Front track
er = car_params.t_r*2; % Rear track
kf = car_params.roll_stiff_f;
kr = car_params.roll_stiff_r;
Ixx = car_params.Ixx;
hcr = car_params.h_cr;
Kr = car_params.K_r;
Cr = car_params.C_r;
hc = car_params.CoG_height;
g = 9.81;


%ODFzL = linear lateral
%OFzE = nonlinear vertical
%OFzL = linear vertical


%State vector
A = zeros(5,5);
H = zeros(5,5);
A = single([1 0 -2*te*(ms/l)*( (lr*hf)/ef + (lf*hr)/er) 0 -2*te*(kf/ef + kr/er);
     0 1 te 0 0;
     0 0 1 0 0;
     0 0 0 1 te;
     0 te*ms*hcr/Ixx 0 te*(ms*g*hcr - Kr)/Ixx  (1+te*(-Cr)/Ixx)]);
%Only use roll rate measurement
%A = single([1 0 -2*te*(ms/l)*( (lr*hf)/ef + (lf*hr)/er) 0 -2*te*(kf/ef + kr/er);
%    0 1 te 0 0;
%    0 0 1 0 0;
%    0 0 0 1 te;
%    0 0 0 0 0]);

% PS: If we measure true linear compensated ay, we dont need to
% adjust with roll angle or gravity. Just double check this.
H = single([0 1 0 0 0;
    0 0 0 1 0;
    0 0 0 0 1;
    1 0 0 0 0]);
%-------------------------------------------------------%
%-------------------------Lateral LKF-------------------%
%-------------------------------------------------------%
persistent firstIteration;
persistent x;
persistent P;

%State Vector: x = [left load transfer , ay_k , der_ay_k , rollAngle, rollRate]
%Measurement vector = [aym, rollAngle, rollRate, left load transfer meas]

%Q = single(diag([1000, 0.1, 0.1, 0.1, 0.1])); % Book parameters
% Notice that last state is weighted very low since there is no process
Q = single(diag([1000, 0.1, 0.1, 0.1, 0.001])); % Book parameters

R = single( diag([0.01 0.01 0.01 100])); % Taken from book

K = single(zeros(5,4));

x_out = single(zeros(5,1));
delta_Fzl = single(0);
if isempty(firstIteration)
    %firstIteration = 2; % Avoid overflow in the register and count 1 again
    %First time the function is called
    %Initialize
    P = single(eye(5));
    x = single(zeros(5,1)); % Also initial value
    x_out = x;
else
	x = A*x; % Prediction of the state
    P = A*P*A' + Q; % Predicted covariance
    
    %Measurement Update
    K = P*H'*inv(H*P*H' + R); % The filter gain
    Y_predicted = H*x; % Predicted measurement
    
    delta_Fzl = -2*(kf/ef + kr/er)*sensor.roll_angle - 2*ms*(sensor.ay/l)*(lr*hf/ef + lf*hr/er);
    Y_meas      = [sensor.ay; sensor.roll_angle; sensor.roll_rate; delta_Fzl];
    
    e = Y_meas - Y_predicted; %Difference between the measurement and predicted measurement 
    x = x + K*e; % Corrected state estimate
    x_out = x;
    P = P - K*H*P;
end

%-------------------------------------------------------%
%-------------------------Vertical Force LKF------------%
%-------------------------------------------------------%
%Assumes superposition principle. Change from LKF to EKF when time
a = te*(-mv*hc)/(2*l);
b = te*(-lr*mv*hc)/(l*ef);
br = te*(-lf*mv*hc)/(l*er);
Av = single([1 0 0 0 0 a 0 b;
            0 1 0 0 0 a 0 -b;
            0 0 1 0 0 -a 0 br;
            0 0 0 1 0 -a 0 -br;
            0 0 0 0 1 te 0 0;
            0 0 0 0 0 1 0 0;
            0 0 0 0 0 0 1 te;
            0 0 0 0 0 0 0 1]);
Hv = single([1 -1 1 -1 0 0 0 0;
            1 1 0 0 0 0 0 0;
            0 0 0 0 1 0 0 0;
            0 0 0 0 0 0 1 0;
            1 1 1 1 0 0 0 0]);
persistent xv;
persistent Pv;


Qv = single(diag([100 100 100 100 0.1 0.001 0.1 0.001])); % From book
Rv = single(diag([0.1 100 0.01 0.01 100])); % Taken from book( VehicleDynest)
Kv = single(zeros(8,5));      % Kalman gain

xv_out = single(zeros(8,1));
Y_measv = single(zeros(5,1));
Y_predictedv = single(zeros(5,1));

%-----------------------------------
%Normal force each tire calculcation
%-----------------------------------
%-----------------------------------
%Normal force each tire calculcation 2
%-----------------------------------
Fz11 = 0.5*mv*(lr*g/l - hc*sensor.ax/l) - mv*(lr*g/l - hc*sensor.ax/l)*hc*sensor.ay/(ef*g);
Fz12 = 0.5*mv*(lr*g/l - hc*sensor.ax/l) + mv*(lr*g/l - hc*sensor.ax/l)*hc*sensor.ay/(ef*g);

Fz21 = 0.5*mv*(lf*g/l + hc*sensor.ax/l) - mv*(lf*g/l + hc*sensor.ax/l)*hc*sensor.ay/(er*g);
Fz22 = 0.5*mv*(lf*g/l + hc*sensor.ax/l) + mv*(lf*g/l + hc*sensor.ax/l)*hc*sensor.ay/(er*g);

FZ = [Fz11; Fz12; Fz21; Fz22];

% Output:
Fz_FL = single(0);
Fz_FR = single(0);
Fz_RL = single(0);
Fz_RR = single(0);



% qf1 = 0.5*mv*(lr*g/l - hc*sensor.a_x/l);
% qf2 = mv*(lr*g/l - hc*sensor.a_x/l)*hc*sensor.a_y/(ef*g);
% Fz11 = qf1 - qf2; % sensor a_y or estimated a_y ????
% Fz12 = qf1 + qf2;
%FzObs = single(mv*(lr*g/l - hc*sensor.ax/l));

normalForces.FL = single(0);
normalForces.FR = single(0);
normalForces.RL = single(0);
normalForces.RR = single(0);

FzObs = single( Fz11 + Fz12);
mxx = single(mv*g/4);
sum_Fz = single(mv*g);
if isempty(firstIteration)
    firstIteration = 2; % Avoid overflow in the register and count 1 again
    %First time the function is called
    %Initialize
    xv = [mxx; mxx; mxx; mxx; 0; 0; 0; 0];
    Pv = single(eye(8));
    xv_out = xv;   
else
	xv = Av*xv; % Prediction of the state
    Pv = Av*Pv*Av' + Qv; % Predicted covariance
    
    %Measurement Update
    Kv = Pv*Hv'/(Hv*Pv*Hv' + Rv); % The filter gain
    Y_predictedv = Hv*xv; % Predicted measurement
    
    Y_measv      = [x(1); FzObs; sensor.ax; x(2); sum_Fz];
    %x(1) = delta_Fzl from other observer
    %x(2) = estimated lateral acceleration compensating for roll angle
    ev = Y_measv - Y_predictedv; %Difference between the measurement and predicted measurement 
    xv = xv + Kv*ev; % Corrected state estimate
    xv_out = xv;
    Pv = Pv - Kv*Hv*Pv;
    normalForces.FL = xv_out(1);
    normalForces.FR = xv_out(2);
    normalForces.RL = xv_out(3);
    normalForces.RR = xv_out(4);
%     Fz_FL = xv_out(1);
%     Fz_FR = xv_out(2);
%     Fz_RL = xv_out(3);
%     Fz_RR = xv_out(4);
    
    
end

== matlab function UnusedModels/Slip ratio ==
  data: SR_Kp output; SR_Ki output; SR_ref output; states input; tractionControl parameter; SR_FL output; SR_FR output; SR_RL output; SR_RR output; speed output
function [SR_Kp, SR_Ki, SR_ref, SR_FL, SR_FR, SR_RL, SR_RR, speed] = slipRatioCalculation(states,tractionControl)
%#codegen
SR_ref = single(tractionControl.Slip_ratio_ref);

SR_FL = single((states.whl_v_FL - states.V_x) / max([0.01, abs(states.whl_v_FL), abs(states.V_x)]));
SR_FR = single((states.whl_v_FR - states.V_x) / max([0.01, abs(states.whl_v_FR), abs(states.V_x)]));
SR_RL = single((states.whl_v_RL - states.V_x) / max([0.01, abs(states.whl_v_RL), abs(states.V_x)]));
SR_RR = single((states.whl_v_RR - states.V_x) / max([0.01, abs(states.whl_v_RR), abs(states.V_x)]));




% GAIN SCHEDULING

%Kp = some function of v_x
%Ki = some function of v_x

SR_Kp = tractionControl.Kp;
SR_Ki = tractionControl.Ki;

speed = states.V_x;
% if (states.V_x < 1) 
%     SR_Kp = single(5);
%     SR_Ki = single(0);
% else
%     SR_Kp = single(5);
%     SR_Ki = single(200);
% end

end

== matlab function UnusedModels/Energy limit Torque Reduction Controller/Energy Limit Control ==
  data: average_power output; states input; energyLimitControl parameter
function average_power  = energyLimitControl(states,energyLimitControl)
%#codegen


%persistent energy;
persistent powerCounter;
persistent firstIteration;
persistent accumulatedTime;
persistent nr_Samples;


if isempty(firstIteration)
    firstIteration = 2; 
    powerCounter = single(0);
    average_power = powerCounter;
    accumulatedTime = single(0);
    
    nr_Samples = single(0);
else
    if (states.power < 0)
        nr_Samples = nr_Samples + single(1);
        powerCounter =  (abs(states.power) + nr_Samples*powerCounter) / (nr_Samples + 1);
        accumulatedTime = accumulatedTime + energyLimitControl.time_since_last_value;
        if (accumulatedTime > energyLimitControl.time_frame)            
            average_power = powerCounter;
        else
            average_power = single(0);
        end 
    else
        nr_Samples = single(0);
        accumulatedTime = single(0);
        powerCounter = single(0);
        average_power = single(0);

    end
end
end

    
    
    

%     
% if (states.effect < 0)
%     energy = energy + abs(energyLimitControl.time_since_last_value*states.effect);
%     accumulated_energy = energy;
% else
%     energy = single(0);
%     accumulated_energy = energy;
% end

== matlab function UnusedModels/FzEstCoupledKalmanFilters ==
  data: normalForces output Bus: normalForces; sensor input Bus: SensorInputs; settings parameter; car_params parameter; x_out output; xv_out output; FZ output; delta_Fzl output
function [normalForces, x_out,xv_out,FZ,delta_Fzl] = normalForceEstimation(sensor, settings,car_params)
%#codegen

te = settings.control_system_sample_time;

ms = car_params.sprung_mass; 
mv = car_params.mass; % Total mass( driver + car)
l = car_params.l; %Wheel base
lr = car_params.l_r;
lf = car_params.l_f;
hr = car_params.h_r;
hf = car_params.h_f;
ef = car_params.t_f*2; % Front track
er = car_params.t_r*2; % Rear track
kf = car_params.roll_stiff_f;
kr = car_params.roll_stiff_r;
Ixx = car_params.Ixx;
hcr = car_params.h_cr;
Kr = car_params.K_r;
Cr = car_params.C_r;
hc = car_params.CoG_height;
g = 9.81;


%ODFzL = linear lateral
%OFzE = nonlinear vertical
%OFzL = linear vertical


%State vector
A = zeros(5,5);
H = zeros(5,5);
A = single([1 0 -2*te*(ms/l)*( (lr*hf)/ef + (lf*hr)/er) 0 -2*te*(kf/ef + kr/er);
     0 1 te 0 0;
     0 0 1 0 0;
     0 0 0 1 te;
     0 te*ms*hcr/Ixx 0 te*(ms*g*hcr - Kr)/Ixx  (1+te*(-Cr)/Ixx)]);
%Only use roll rate measurement
%A = single([1 0 -2*te*(ms/l)*( (lr*hf)/ef + (lf*hr)/er) 0 -2*te*(kf/ef + kr/er);
%    0 1 te 0 0;
%    0 0 1 0 0;
%    0 0 0 1 te;
%    0 0 0 0 0]);

% PS: If we measure true linear compensated ay, we dont need to
% adjust with roll angle or gravity. Just double check this.
H = single([0 1 0 0 0;
    0 0 0 1 0;
    0 0 0 0 1;
    1 0 0 0 0]);
%-------------------------------------------------------%
%-------------------------Lateral LKF-------------------%
%-------------------------------------------------------%
persistent firstIteration;
persistent x;
persistent P;

%State Vector: x = [left load transfer , ay_k , der_ay_k , rollAngle, rollRate]
%Measurement vector = [aym, rollAngle, rollRate, left load transfer meas]


% Notice that last state is weighted very low since there is no process
%Q = single(diag([1000, 0.1, 0.1, 0.1, 0.1])); % Book parameters
%R = single( diag([0.01 0.01 0.01 100])); % Taken from book

Q = single(diag([1000, 10, 10, 1000000, 1000000]));
R = single( diag([0.01 0.01 0.01 100])); 
K = single(zeros(5,4));

x_out = single(zeros(5,1));
delta_Fzl = single(0);
if isempty(firstIteration)
    %firstIteration = 2; % Avoid overflow in the register and count 1 again
    %First time the function is called
    %Initialize
    P = single(eye(5));
    x = single(zeros(5,1)); % Also initial value
    x_out = x;
else
	x = A*x; % Prediction of the state
    P = A*P*A' + Q; % Predicted covariance
    
    %Measurement Update
    K = P*H'*inv(H*P*H' + R); % The filter gain
    Y_predicted = H*x; % Predicted measurement
    
    delta_Fzl = -2*(kf/ef + kr/er)*sensor.roll_angle - 2*ms*(sensor.ay/l)*(lr*hf/ef + lf*hr/er);
    Y_meas      = [sensor.ay; sensor.roll_angle; sensor.roll_rate; delta_Fzl];
    
    e = Y_meas - Y_predicted; %Difference between the measurement and predicted measurement 
    x = x + K*e; % Corrected state estimate
    x_out = x;
    P = P - K*H*P;
end

%-------------------------------------------------------%
%-------------------------Vertical Force LKF------------%
%-------------------------------------------------------%
%Assumes superposition principle. Change from LKF to EKF when time
a = te*(-mv*hc)/(2*l);
b = te*(-lr*mv*hc)/(l*ef);
br = te*(-lf*mv*hc)/(l*er);
Av = single([1 0 0 0 0 a 0 b;
            0 1 0 0 0 a 0 -b;
            0 0 1 0 0 -a 0 br;
            0 0 0 1 0 -a 0 -br;
            0 0 0 0 1 te 0 0;
            0 0 0 0 0 1 0 0;
            0 0 0 0 0 0 1 te;
            0 0 0 0 0 0 0 1]);
Hv = single([1 -1 1 -1 0 0 0 0;
            1 1 0 0 0 0 0 0;
            0 0 0 0 1 0 0 0;
            0 0 0 0 0 0 1 0;
            1 1 1 1 0 0 0 0]);
%EKF constants
a1 = hc*mv/(2*l);
b1 = mv*lr*hc/(l*ef);
c1 = mv*(hc^2)/(l*ef*g);
d1 = mv*(hc^2)/(l*ef*g);
a2 = hc*mv/(2*l);
b2 = mv*lr*hc/(l*ef);
c2 = mv*(hc^2)/(l*er*g);
d2 = mv*(hc^2)/(l*er*g);

persistent xv;
persistent Pv;

%state = FzFL, FzFR, FzRL,FzRR, ax, ax_der, ay, ay_der
%Meas = sumLateral, FzFL+FzFR, ax, ay, sumFz

%Qv = single(diag([100 100 100 100 0.1 0.001 0.1 0.001])); % From book
%Rv = single(diag([0.1 100 0.01 0.01 100])); % Taken from book( VehicleDynest)
Qv = single(diag([0.000100 0.000100 0.000100 0.000100 0.1 0.001 0.1 0.001])); % From book
Rv = single(diag([0.001 0.001 0.0001 0.000001 100])); % Taken from book( VehicleDynest)


Kv = single(zeros(8,5));      % Kalman gain
xv_out = single(zeros(8,1));
Y_measv = single(zeros(5,1));
Y_predictedv = single(zeros(5,1));

%-----------------------------------
%Normal force each tire calculcation
%-----------------------------------
%-----------------------------------
%Normal force each tire calculcation 2
%-----------------------------------
Fz11 = 0.5*mv*(lr*g/l - hc*sensor.ax/l) - mv*(lr*g/l - hc*sensor.ax/l)*hc*sensor.ay/(ef*g);
Fz12 = 0.5*mv*(lr*g/l - hc*sensor.ax/l) + mv*(lr*g/l - hc*sensor.ax/l)*hc*sensor.ay/(ef*g);

Fz21 = 0.5*mv*(lf*g/l + hc*sensor.ax/l) - mv*(lf*g/l + hc*sensor.ax/l)*hc*sensor.ay/(er*g);
Fz22 = 0.5*mv*(lf*g/l + hc*sensor.ax/l) + mv*(lf*g/l + hc*sensor.ax/l)*hc*sensor.ay/(er*g);

FZ = [Fz11; Fz12; Fz21; Fz22];

% Output:
Fz_FL = single(0);
Fz_FR = single(0);
Fz_RL = single(0);
Fz_RR = single(0);



% qf1 = 0.5*mv*(lr*g/l - hc*sensor.a_x/l);
% qf2 = mv*(lr*g/l - hc*sensor.a_x/l)*hc*sensor.a_y/(ef*g);
% Fz11 = qf1 - qf2; % sensor a_y or estimated a_y ????
% Fz12 = qf1 + qf2;
%FzObs = single(mv*(lr*g/l - hc*sensor.ax/l));

normalForces.FL = single(0);
normalForces.FR = single(0);
normalForces.RL = single(0);
normalForces.RR = single(0);

FzObs = single( Fz11 + Fz12);
mxx = single(mv*g/4);
sum_Fz = single(mv*g);
if isempty(firstIteration)
    firstIteration = 2; % Avoid overflow in the register and count 1 again
    %First time the function is called
    %Initialize
    xv = [mxx; mxx; mxx; mxx; 0; 0; 0; 0];
    Pv = single(eye(8));
    xv_out = xv;   
else
    % Solve f(xk-1)
    J = [1, 0, 0, 0, (c1*te*xv(8)), (-te*(a1 - d1*xv(7))), (d1*te*xv(6)),   (-te*(b1 - c1*xv(5)));
         0, 1, 0, 0, (-c1*te*xv(8)), (-te*(a1 + d1*xv(7))), (-d1*te*xv(6)), (-te*(b1 - c1*xv(5)));
         0, 0, 1, 0, (-c2*te*xv(8)), (te*(a2 - d2*xv(7))), (-d2*te*xv(6)),  (-te*(b2 + c2*xv(5)));
         0, 0, 0, 1, (c2*te*xv(8)), (te*(a2  + d2*xv(7))), (d2*te*xv(6)),   (te*(b2  + c2*xv(5)));
         0, 0, 0, 0,    1,              te,                     0,                  0;
         0, 0, 0, 0,    0,              1,                      0,                  0;
         0, 0, 0, 0,    0,              0,                      1,                  te;
         0, 0, 0, 0,    0,              0,                      0,                  1];
    
    xv = [ (xv(1) + te*(-a1*xv(6) - b1*xv(8) + c1*xv(5)*xv(8) + d1*xv(6)*xv(7)));
           (xv(2) + te*(-a1*xv(6) + b1*xv(8) - c1*xv(5)*xv(8) - d1*xv(6)*xv(7)));
           (xv(3) + te*(a2*xv(6)  - b2*xv(8) - c2*xv(5)*xv(8) - d2*xv(6)*xv(7)));
           (xv(4) + te*(a2*xv(6)  + b2*xv(8) + c1*xv(5)*xv(8) + d1*xv(6)*xv(7)));
           (xv(5) + te*xv(6));
           (xv(6));
           (xv(7) + te*xv(8));
           (xv(8))];
    
    Pv = J*Pv*J' + Qv;
    
    %Measurement Update
    Kv = Pv*Hv'/(Hv*Pv*Hv' + Rv); % The filter gain
    Y_predictedv = Hv*xv; % Predicted measurement
    
    Y_measv      = [x(1); FzObs; sensor.ax; x(2); sum_Fz];

    ev = Y_measv - Y_predictedv; %Difference between the measurement and predicted measurement 
    xv = xv + Kv*ev; % Corrected state estimate
    xv_out = xv;
    Pv = Pv - Kv*Hv*Pv;
    normalForces.FL = xv_out(1);
    normalForces.FR = xv_out(2);
    normalForces.RL = xv_out(3);
    normalForces.RR = xv_out(4);
%     Fz_FL = xv_out(1);
%     Fz_FR = xv_out(2);
%     Fz_RL = xv_out(3);
%     Fz_RR = xv_out(4);
    
    
end

== matlab function UnusedModels/Coasting KERS at 0 torque request/MATLAB Function ==
  data: active output; states input; Ti_coast output Bus: Ti_lim; settings parameter
function [active,Ti_coast] = coastingKERS(states,settings)
%#codegen


active = int32(1);

% if ( (states.V_x > 5) &&...
%      (states.Input_throttle < settings.throttle_not_active_threshold) &&...
%      (states.KERS_pos < settings.KERS_not_active_treshold) )  
%     active = int32(-1); % Active
% else
%     active = int32(1);
% end




Ti_lim_struct = struct;
Ti_lim_struct.FL = -settings.max_motor_torque*4*settings.coasting_KERS_percent;
Ti_lim_struct.FR = -settings.max_motor_torque*4*settings.coasting_KERS_percent;
Ti_lim_struct.RL = -settings.max_motor_torque*4*settings.coasting_KERS_percent;
Ti_lim_struct.RR = -settings.max_motor_torque*4*settings.coasting_KERS_percent;

Ti_coast = Ti_lim_struct;

end
